simulink model "VCU_SW"  (R2020b)
settings: Solver=FixedStepDiscrete  StartTime=0.0  StopTime=inf  FixedStep=1e-2  RelTol=1e-3
PreLoadFcn:
  | RTWConfigurationCB('preloadfcn', bdroot);
InitFcn:
  | loadvar_ttc500
undefined symbols (not defined in the file or in its folder): BrkPedalTypes, CabMovModeTypes, cFuseTempSensAcc_X, cFuseTempSensAcc_Y, cFuseTempSensVal_X, cFuseTempSensVal_Y, cTMSTempSensVal_X, cTMSTempSensVal_Y, cTransferCaseSpeedRatio, diag_state, DoorsPositionTypes, dP_filter_Y, DriverOccClassSystemTypes, ErrorValueTypes, fatal_error_callback, IO_ADC_NO_RANGE, LadderStatusTypes, pAnalogCabRotSensAcc, pAnalogCabRotSensMaxVolt, pAnalogCabRotSensMinVolt, pAnalogCabRotSensRange, pAnalogCabRotSensZeroVolt, pBrkActivePress, pCabTiltSensAcc, pCabTiltSensMaxCur, pCabTiltSensMinCur, pDistanceCorrection, pECANManual_BPNEnable, pECANManual_BPNEnabler_Flag, pFilterSensAccRes, pHDirMaxDiffFrq, pHDirSensHighLvl, pHDirSensLowLvl, pMainGearRatio, pMaxFilterSensRes, pMaxFirstPedalSensValue, pMaxFuseTempSensRes, pMaxPressLoss, pMaxPressSensCurrent, pMaxPressValue, pMaxPressValueHydMotAndPump, pMaxPressValueParkDrain, pMaxSecondPedalSensValue, pMaxTempSensVoltage, pMaxTempValue, pMaxTMSTempSensRes, pMinFilterSensRes, pMinFirstPedalSensValue, pMinFuseTempSensRes, pMinPressLoss, pMinPressSensCurrent, pMinPressValue, pMinSecondPedalSensValue, pMinTempSensVoltage, pMinTempValue, pMinTMSTempSensRes, pMotorRingTeethNum, pPedalSensAccuracyPct, pPedalSensAccuracyVolt, pPressLossTreshhold ... (+20)
libraries: TTlibrary x271, canmsglib x128, simulink x88
(part 7 of 17)

== system VCU_SW/OutputLayer/OutputInterfaces/exDigitalOutput/SetDO1000msec ==
  function : TriggerPort  TriggerType=function-call  VariantControl=Variant
  Constant50 : Constant  OutDataTypeStr=uint8
  Constant51 : Constant  Value=0  OutDataTypeStr=uint8
  Data Store Read15 : DataStoreRead  DataStoreName=OutputInterfaceData  DataStoreElements=OutputInterfaceData.DO.lowBrakeFluidSensSupply
  Data Store Read61 : DataStoreRead  DataStoreName=ManualOutputInterfaceData  DataStoreElements=ManualOutputInterfaceData.DO_Man.man_lowBrakeFluidSensSupply
  Data Type Conversion25 : DataTypeConversion  OutDataTypeStr=boolean
  Function Caller16 : FunctionCaller  FunctionPrototype=rawValue = convDIOStsTypeToNum(enumValue)  InputArgumentSpecifications=<Enter example>  OutputArgumentSpecifications=<Enter example>
  Logical Operator25 : Logic  Operator=OR  AllPortsSameDT=off  OutDataTypeStr=boolean
  Multiport Switch25 : MultiPortSwitch  DataPortOrder=Zero-based contiguous  Inputs=2  zeroidx=on
  Relational Operator50 : RelationalOperator  Operator===  OutDataTypeStr=boolean  RndMeth=Simplest
  Relational Operator51 : RelationalOperator  Operator===  OutDataTypeStr=boolean  RndMeth=Simplest
  Terminator10 : Terminator
  setDigitalOutputValue16 : TTlibrary/DIO/setDigitalOutputValue  do_channel=IO_DO_41  diagnostic=FALSE  safety_conf=off  low_side_safety_channel=IO_DO_08  io_error=on  sample_time=-1
      settings: SourceProductName=TT control 500 series
  wires:
  Data Type Conversion25/1 -> Multiport Switch25/3
  Constant51/1 -> Relational Operator50/2
  Relational Operator50/1 -> Logical Operator25/2
  Multiport Switch25/1 -> setDigitalOutputValue16/1
  Logical Operator25/1 -> Multiport Switch25/1
  Data Store Read15/1 -> Function Caller16/1
  Relational Operator51/1 -> Logical Operator25/1
  Data Store Read61/1 -> Relational Operator51/1, Relational Operator50/1, Data Type Conversion25/1
  setDigitalOutputValue16/1 -> Terminator10/1
  Constant50/1 -> Relational Operator51/2
  Function Caller16/1 -> Multiport Switch25/2

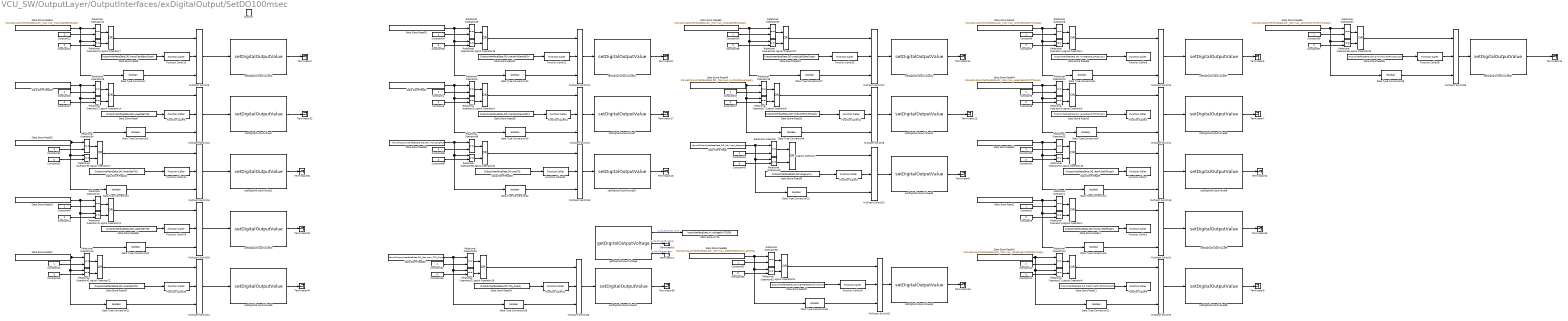
== system VCU_SW/OutputLayer/OutputInterfaces/exDigitalOutput/SetDO100msec ==
  function : TriggerPort  TriggerType=function-call  VariantControl=Variant
  Constant{2,4,6,8,10,12,16,26,30,32,34,40,42,44,52,54,56,62,68} (19 alike) : Constant  OutDataTypeStr=uint8
  Constant{3,5,7,9,11,13,17,27,31,33,35,41,43,45,53,55,57,63,69} (19 alike) : Constant  Value=0  OutDataTypeStr=uint8
  Data Store Read : DataStoreRead  DataStoreName=ManualOutputInterfaceData  DataStoreElements=ManualOutputInterfaceData.DO_Man.man_diagLamp
  Data Store Read10 : DataStoreRead  DataStoreName=OutputInterfaceData  DataStoreElements=OutputInterfaceData.DO.upperGearDistrTCSupply
  Data Store Read11 : DataStoreRead  DataStoreName=OutputInterfaceData  DataStoreElements=OutputInterfaceData.DO.disablingFrontDrDistrSupply
  Data Store Read12 : DataStoreRead  DataStoreName=OutputInterfaceData  DataStoreElements=OutputInterfaceData.DO.starterSolenoidCtrl
  Data Store Read14 : DataStoreRead  DataStoreName=OutputInterfaceData  DataStoreElements=OutputInterfaceData.DO.frontAxleDifSupply
  Data Store Read19 : DataStoreRead  DataStoreName=ManualOutputInterfaceData  DataStoreElements=ManualOutputInterfaceData.DO_Man.man_upperGenT15
  Data Store Read2 : DataStoreRead  DataStoreName=ManualOutputInterfaceData  DataStoreElements=ManualOutputInterfaceData.DO_Man.man_frontAxleDifSupply
  Data Store Read22 : DataStoreRead  DataStoreName=OutputInterfaceData  DataStoreElements=OutputInterfaceData.DO.lowerGenT15
  Data Store Read23 : DataStoreRead  DataStoreName=OutputInterfaceData  DataStoreElements=OutputInterfaceData.DO.stopLightSensSupply
  Data Store Read24 : DataStoreRead  DataStoreName=OutputInterfaceData  DataStoreElements=OutputInterfaceData.DO.lowerGenT15
  Data Store Read27 : DataStoreRead  DataStoreName=OutputInterfaceData  DataStoreElements=OutputInterfaceData.DO.engPreheaterActivationSig
  Data Store Read28 : DataStoreRead  DataStoreName=OutputInterfaceData  DataStoreElements=OutputInterfaceData.DO.starterSolenoidCtrl
  Data Store Read3 : DataStoreRead  DataStoreName=ManualOutputInterfaceData  DataStoreElements=ManualOutputInterfaceData.DO_Man.man_lowerGearDistrTCSupply
  Data Store Read31 : DataStoreRead  DataStoreName=OutputInterfaceData  DataStoreElements=OutputInterfaceData.DO.HydCANPowerSupply
  Data Store Read32 : DataStoreRead  DataStoreName=OutputInterfaceData  DataStoreElements=OutputInterfaceData.DO.engT15
  Data Store Read34 : DataStoreRead  DataStoreName=OutputInterfaceData  DataStoreElements=OutputInterfaceData.DO.T15_Supply
  Data Store Read35 : DataStoreRead  DataStoreName=OutputInterfaceData  DataStoreElements=OutputInterfaceData.DO.IgnitionSwitchPowerSupply
  Data Store Read36 : DataStoreRead  DataStoreName=OutputInterfaceData  DataStoreElements=OutputInterfaceData.DO.diagLamp
  Data Store Read39 : DataStoreRead  DataStoreName=OutputInterfaceData  DataStoreElements=OutputInterfaceData.DO.lowerGearDistrTCSupply
  Data Store Read4 : DataStoreRead  DataStoreName=ManualOutputInterfaceData  DataStoreElements=ManualOutputInterfaceData.DO_Man.man_starterSolenoidCtrl
  Data Store Read40 : DataStoreRead  DataStoreName=ManualOutputInterfaceData  DataStoreElements=ManualOutputInterfaceData.DO_Man.man_upperGearDistrTCSupply
  Data Store Read41 : DataStoreRead  DataStoreName=ManualOutputInterfaceData  DataStoreElements=ManualOutputInterfaceData.DO_Man.man_disablingFrontDrDistrSupply
  Data Store Read42 : DataStoreRead  DataStoreName=ManualOutputInterfaceData  DataStoreElements=ManualOutputInterfaceData.DO_Man.man_transCaseSensSupply
  Data Store Read44 : DataStoreRead  DataStoreName=ManualOutputInterfaceData  DataStoreElements=ManualOutputInterfaceData.DO_Man.man_HydCANPowerSupply
  Data Store Read49 : DataStoreRead  DataStoreName=ManualOutputInterfaceData  DataStoreElements=ManualOutputInterfaceData.DO_Man.man_upperGenT15
  Data Store Read5 : DataStoreRead  DataStoreName=OutputInterfaceData  DataStoreElements=OutputInterfaceData.DO.transCaseSensSupply
  Data Store Read51 : DataStoreRead  DataStoreName=ManualOutputInterfaceData  DataStoreElements=ManualOutputInterfaceData.DO_Man.man_rearAxleDifSupply
  Data Store Read52 : DataStoreRead  DataStoreName=ManualOutputInterfaceData  DataStoreElements=ManualOutputInterfaceData.DO_Man.man_lowerGenT15
  Data Store Read53 : DataStoreRead  DataStoreName=ManualOutputInterfaceData  DataStoreElements=ManualOutputInterfaceData.DO_Man.man_starterSolenoidCtrl
  Data Store Read56 : DataStoreRead  DataStoreName=OutputInterfaceData  DataStoreElements=OutputInterfaceData.DO.upperGenT15
  Data Store Read57 : DataStoreRead  DataStoreName=ManualOutputInterfaceData  DataStoreElements=ManualOutputInterfaceData.DO_Man.man_lowerGenT15
  Data Store Read62 : DataStoreRead  DataStoreName=ManualOutputInterfaceData  DataStoreElements=ManualOutputInterfaceData.DO_Man.man_T15_Supply
  Data Store Read63 : DataStoreRead  DataStoreName=ManualOutputInterfaceData  DataStoreElements=ManualOutputInterfaceData.DO_Man.man_stopLightSensSupply
  Data Store Read64 : DataStoreRead  DataStoreName=ManualOutputInterfaceData  DataStoreElements=ManualOutputInterfaceData.DO_Man.man_IgnitionSwitchPowerSupply
  Data Store Read66 : DataStoreRead  DataStoreName=ManualOutputInterfaceData  DataStoreElements=ManualOutputInterfaceData.DO_Man.man_engPreheaterActivationSig
  Data Store Read69 : DataStoreRead  DataStoreName=ManualOutputInterfaceData  DataStoreElements=ManualOutputInterfaceData.DO_Man.man_engT15
  Data Store Read7 : DataStoreRead  DataStoreName=OutputInterfaceData  DataStoreElements=OutputInterfaceData.DO.upperGenT15
  Data Store Read9 : DataStoreRead  DataStoreName=OutputInterfaceData  DataStoreElements=OutputInterfaceData.DO.rearAxleDifSupply
  Data Store Write : DataStoreWrite  DataStoreName=InputInterfaceData  DataStoreElements=InputInterfaceData.AI.voltageOnT15DO
  Data Type Conversion{,2,4..9,12..13,19..22,26..28,31,34} (19 alike) : DataTypeConversion  OutDataTypeStr=boolean
  Function Caller{1..5,7,9..13,20..21,24,26,29..31,35} (19 alike) : FunctionCaller  FunctionPrototype=rawValue = convDIOStsTypeToNum(enumValue)  InputArgumentSpecifications=<Enter example>  OutputArgumentSpecifications=<Enter example>
  Logical Operator{,1,3..7,9,14,16..18,21..22,26..28,31,34} (19 alike) : Logic  Operator=OR  AllPortsSameDT=off  OutDataTypeStr=boolean
  Multiport Switch{1..6,8,13,15..17,20..21,26..28,31,34} (18 alike) : MultiPortSwitch  DataPortOrder=Zero-based contiguous  Inputs=2  zeroidx=on
  Multiport Switch22 : MultiPortSwitch  DataPortOrder=Zero-based contiguous  Inputs=2  DiagnosticForDefault=None  zeroidx=on
  Relational Operator{,1,4..14,17..18,27..28,31..36,41..45,52..57,62..63,68..69} (38 alike) : RelationalOperator  Operator===  OutDataTypeStr=boolean  RndMeth=Simplest
  Terminator{1..3,5..9,13,16..17,32,34..36,38..39,42..44,48} (21 alike) : Terminator
  getDigitalOutputVoltage : TTlibrary/DIO/getDigitalOutputVoltage  do_channel=IO_DO_03  io_error=on  sample_time=-1
      settings: SourceProductName=TT control 500 series
  setDigitalOutputValue10 : TTlibrary/DIO/setDigitalOutputValue  do_channel=IO_DO_39  diagnostic=FALSE  safety_conf=off  low_side_safety_channel=IO_DO_08  io_error=on  sample_time=-1
      settings: SourceProductName=TT control 500 series
  setDigitalOutputValue11 : TTlibrary/DIO/setDigitalOutputValue  do_channel=IO_DO_20  diagnostic=FALSE  safety_conf=off  low_side_safety_channel=IO_DO_08  io_error=on  sample_time=-1
      settings: SourceProductName=TT control 500 series
  setDigitalOutputValue12 : TTlibrary/DIO/setDigitalOutputValue  do_channel=IO_DO_06  diagnostic=FALSE  safety_conf=off  low_side_safety_channel=IO_DO_08  io_error=on  sample_time=-1
      settings: SourceProductName=TT control 500 series
  setDigitalOutputValue13 : TTlibrary/DIO/setDigitalOutputValue  do_channel=IO_DO_45  diagnostic=FALSE  safety_conf=off  low_side_safety_channel=IO_DO_08  io_error=on  sample_time=-1
      settings: SourceProductName=TT control 500 series
  setDigitalOutputValue20 : TTlibrary/DIO/setDigitalOutputValue  do_channel=IO_DO_51  diagnostic=FALSE  safety_conf=off  low_side_safety_channel=IO_DO_08  io_error=on  sample_time=-1
      settings: SourceProductName=TT control 500 series
  setDigitalOutputValue21 : TTlibrary/DIO/setDigitalOutputValue  do_channel=IO_DO_03  diagnostic=FALSE  safety_conf=off  low_side_safety_channel=IO_DO_08  io_error=on  sample_time=-1
      settings: SourceProductName=TT control 500 series
  setDigitalOutputValue24 : TTlibrary/DIO/setDigitalOutputValue  do_channel=IO_DO_33  diagnostic=FALSE  safety_conf=off  low_side_safety_channel=IO_DO_08  io_error=on  sample_time=-1
      settings: SourceProductName=TT control 500 series
  setDigitalOutputValue25 : TTlibrary/DIO/setDigitalOutputValue  do_channel=IO_DO_07  diagnostic=FALSE  safety_conf=off  low_side_safety_channel=IO_DO_08  io_error=on  sample_time=-1
      settings: SourceProductName=TT control 500 series
  setDigitalOutputValue26 : TTlibrary/DIO/setDigitalOutputValue  do_channel=IO_DO_21  diagnostic=FALSE  safety_conf=off  low_side_safety_channel=IO_DO_08  io_error=on  sample_time=-1
      settings: SourceProductName=TT control 500 series
  setDigitalOutputValue30 : TTlibrary/DIO/setDigitalOutputValue  do_channel=IO_DO_24  diagnostic=FALSE  safety_conf=off  low_side_safety_channel=IO_DO_08  io_error=on  sample_time=-1
      settings: SourceProductName=TT control 500 series
  setDigitalOutputValue35 : TTlibrary/DIO/setDigitalOutputValue  do_channel=IO_DO_42  diagnostic=FALSE  safety_conf=off  low_side_safety_channel=IO_DO_08  io_error=on  sample_time=-1
      settings: SourceProductName=TT control 500 series
  setDigitalOutputValue36 : TTlibrary/DIO/setDigitalOutputValue  do_channel=IO_DO_34  diagnostic=FALSE  safety_conf=off  low_side_safety_channel=IO_DO_08  io_error=on  sample_time=-1
      settings: SourceProductName=TT control 500 series
  setDigitalOutputValue37 : TTlibrary/DIO/setDigitalOutputValue  do_channel=IO_DO_23  diagnostic=FALSE  safety_conf=off  low_side_safety_channel=IO_DO_08  io_error=on  sample_time=-1
      settings: SourceProductName=TT control 500 series
  setDigitalOutputValue38 : TTlibrary/DIO/setDigitalOutputValue  do_channel=IO_DO_37  diagnostic=FALSE  safety_conf=off  low_side_safety_channel=IO_DO_08  io_error=on  sample_time=-1
      settings: SourceProductName=TT control 500 series
  setDigitalOutputValue39 : TTlibrary/DIO/setDigitalOutputValue  do_channel=IO_DO_25  diagnostic=FALSE  safety_conf=off  low_side_safety_channel=IO_DO_08  io_error=on  sample_time=-1
      settings: SourceProductName=TT control 500 series
  setDigitalOutputValue4 : TTlibrary/DIO/setDigitalOutputValue  do_channel=IO_DO_50  diagnostic=FALSE  safety_conf=off  low_side_safety_channel=IO_DO_08  io_error=on  sample_time=-1
      settings: SourceProductName=TT control 500 series
  setDigitalOutputValue7 : TTlibrary/DIO/setDigitalOutputValue  do_channel=IO_DO_38  diagnostic=FALSE  safety_conf=off  low_side_safety_channel=IO_DO_08  io_error=on  sample_time=-1
      settings: SourceProductName=TT control 500 series
  setDigitalOutputValue8 : TTlibrary/DIO/setDigitalOutputValue  do_channel=IO_DO_18  diagnostic=FALSE  safety_conf=off  low_side_safety_channel=IO_DO_08  io_error=on  sample_time=-1
      settings: SourceProductName=TT control 500 series
  setDigitalOutputValue9 : TTlibrary/DIO/setDigitalOutputValue  do_channel=IO_DO_32  diagnostic=FALSE  safety_conf=off  low_side_safety_channel=IO_DO_08  io_error=on  sample_time=-1
      settings: SourceProductName=TT control 500 series
  wires:
  Logical Operator7/1 -> Multiport Switch6/1
  Multiport Switch6/1 -> setDigitalOutputValue13/1
  Function Caller13/1 -> Multiport Switch6/2
  Data Store Read5/1 -> Function Caller13/1
  Data Type Conversion/1 -> Multiport Switch6/3
  Relational Operator13/1 -> Logical Operator7/2
  setDigitalOutputValue13/1 -> Terminator2/1
  Data Store Read42/1 -> Relational Operator14/1, Relational Operator13/1, Data Type Conversion/1
  Constant13/1 -> Relational Operator13/2
  Constant12/1 -> Relational Operator14/2
  Relational Operator14/1 -> Logical Operator7/1
  Function Caller5/1 -> Multiport Switch13/2
  Constant27/1 -> Relational Operator27/2
  setDigitalOutputValue4/1 -> Terminator32/1
  Data Store Read52/1 -> Relational Operator34/1, Relational Operator33/1, Data Type Conversion7/1
  Relational Operator27/1 -> Logical Operator14/2
  Relational Operator34/1 -> Logical Operator17/1
  Constant32/1 -> Relational Operator34/2
  Constant26/1 -> Relational Operator28/2
  Relational Operator33/1 -> Logical Operator17/2
  Data Store Read49/1 -> Relational Operator28/1, Relational Operator27/1, Data Type Conversion2/1
  Function Caller10/1 -> Multiport Switch16/2
  Logical Operator17/1 -> Multiport Switch16/1
  Data Store Read22/1 -> Function Caller10/1
  Relational Operator28/1 -> Logical Operator14/1
  Data Type Conversion7/1 -> Multiport Switch16/3
  Constant33/1 -> Relational Operator33/2
  Multiport Switch13/1 -> setDigitalOutputValue4/1
  Logical Operator14/1 -> Multiport Switch13/1
  setDigitalOutputValue11/1 -> Terminator36/1
  Data Store Read7/1 -> Function Caller5/1
  Multiport Switch16/1 -> setDigitalOutputValue11/1
  Data Type Conversion2/1 -> Multiport Switch13/3
  Constant40/1 -> Relational Operator42/2
  Logical Operator21/1 -> Multiport Switch20/1
  Relational Operator42/1 -> Logical Operator21/1
  Relational Operator41/1 -> Logical Operator21/2
  Constant41/1 -> Relational Operator41/2
  Data Store Read19/1 -> Relational Operator42/1, Relational Operator41/1, Data Type Conversion20/1
  Multiport Switch20/1 -> setDigitalOutputValue20/1
  setDigitalOutputValue20/1 -> Terminator38/1
  Data Store Read56/1 -> Function Caller24/1
  Function Caller24/1 -> Multiport Switch20/2
  Data Type Conversion20/1 -> Multiport Switch20/3
  Relational Operator43/1 -> Logical Operator22/2
  Data Store Read24/1 -> Function Caller29/1
  Relational Operator44/1 -> Logical Operator22/1
  Multiport Switch21/1 -> setDigitalOutputValue26/1
  Data Type Conversion21/1 -> Multiport Switch21/3
  setDigitalOutputValue26/1 -> Terminator44/1
  Logical Operator22/1 -> Multiport Switch21/1
  Constant42/1 -> Relational Operator44/2
  Data Store Read57/1 -> Relational Operator44/1, Relational Operator43/1, Data Type Conversion21/1
  Constant43/1 -> Relational Operator43/2
  Function Caller29/1 -> Multiport Switch21/2
  Data Store Read62/1 -> Relational Operator53/1, Relational Operator52/1, Data Type Conversion26/1
  setDigitalOutputValue10/1 -> Terminator9/1
  Multiport Switch34/1 -> setDigitalOutputValue35/1
  Relational Operator36/1 -> Logical Operator18/1
  getDigitalOutputVoltage/3 -> Terminator1/1  "io_do_03_amp_error"
  Function Caller31/1 -> Multiport Switch2/2
  Data Type Conversion12/1 -> Multiport Switch17/3
  Data Store Read32/1 -> Function Caller35/1
  Logical Operator26/1 -> Multiport Switch26/1
  Multiport Switch17/1 -> setDigitalOutputValue10/1
  Data Store Read34/1 -> Function Caller21/1
  setDigitalOutputValue7/1 -> Terminator17/1
  Data Store Read12/1 -> Function Caller11/1
  Logical Operator34/1 -> Multiport Switch34/1
  Constant68/1 -> Relational Operator69/2
  Constant52/1 -> Relational Operator53/2
  Relational Operator5/1 -> Logical Operator3/2
  Function Caller11/1 -> Multiport Switch17/2
  Relational Operator52/1 -> Logical Operator26/2
  Constant53/1 -> Relational Operator52/2
  Relational Operator35/1 -> Logical Operator18/2
  Logical Operator18/1 -> Multiport Switch17/1
  getDigitalOutputVoltage/1 -> Data Store Write/1  "io_do_03_amp_value"
  setDigitalOutputValue21/1 -> Terminator39/1
  Relational Operator68/1 -> Logical Operator34/2
  Logical Operator3/1 -> Multiport Switch2/1
  Data Store Read69/1 -> Relational Operator69/1, Relational Operator68/1, Data Type Conversion34/1
  Data Store Read4/1 -> Relational Operator6/1, Relational Operator5/1, Data Type Conversion19/1
  Constant69/1 -> Relational Operator68/2
  Multiport Switch2/1 -> setDigitalOutputValue7/1
  getDigitalOutputVoltage/2 -> Terminator3/1  "io_do_03_amp_update"
  setDigitalOutputValue35/1 -> Terminator48/1
  Function Caller21/1 -> Multiport Switch26/2
  Data Type Conversion34/1 -> Multiport Switch34/3
  Data Store Read28/1 -> Function Caller31/1
  Multiport Switch26/1 -> setDigitalOutputValue21/1
  Relational Operator69/1 -> Logical Operator34/1
  Data Store Read53/1 -> Relational Operator36/1, Relational Operator35/1, Data Type Conversion12/1
  Data Type Conversion26/1 -> Multiport Switch26/3
  Constant5/1 -> Relational Operator5/2
  Constant4/1 -> Relational Operator6/2
  Data Type Conversion19/1 -> Multiport Switch2/3
  Relational Operator6/1 -> Logical Operator3/1
  Constant35/1 -> Relational Operator35/2
  Constant34/1 -> Relational Operator36/2
  Relational Operator53/1 -> Logical Operator26/1
  Function Caller35/1 -> Multiport Switch34/2
  Function Caller20/1 -> Multiport Switch27/2
  Data Type Conversion27/1 -> Multiport Switch27/3
  Constant54/1 -> Relational Operator55/2
  Logical Operator27/1 -> Multiport Switch27/1
  Constant55/1 -> Relational Operator54/2
  Relational Operator55/1 -> Logical Operator27/1
  Multiport Switch27/1 -> setDigitalOutputValue24/1
  setDigitalOutputValue24/1 -> Terminator42/1
  Data Store Read63/1 -> Relational Operator55/1, Relational Operator54/1, Data Type Conversion27/1
  Data Store Read23/1 -> Function Caller20/1
  Relational Operator54/1 -> Logical Operator27/2
  Data Store Read40/1 -> Relational Operator10/1, Relational Operator9/1, Data Type Conversion9/1
  setDigitalOutputValue37/1 -> Terminator5/1
  Data Type Conversion8/1 -> Multiport Switch3/3
  Constant11/1 -> Relational Operator11/2
  Relational Operator1/1 -> Logical Operator1/2
  Constant10/1 -> Relational Operator12/2
  Relational Operator31/1 -> Logical Operator16/2
  Data Store Read51/1 -> Relational Operator32/1, Relational Operator31/1, Data Type Conversion4/1
  Logical Operator6/1 -> Multiport Switch5/1
  Multiport Switch15/1 -> setDigitalOutputValue8/1
  setDigitalOutputValue8/1 -> Terminator34/1
  Relational Operator12/1 -> Logical Operator6/1
  setDigitalOutputValue9/1 -> Terminator35/1
  Logical Operator1/1 -> Multiport Switch1/1
  Constant3/1 -> Relational Operator1/2
  Multiport Switch5/1 -> setDigitalOutputValue39/1
  Constant31/1 -> Relational Operator31/2
  Logical Operator16/1 -> Multiport Switch15/1
  Data Store Read9/1 -> Function Caller7/1
  Relational Operator4/1 -> Logical Operator1/1
  Data Type Conversion4/1 -> Multiport Switch15/3
  Constant2/1 -> Relational Operator4/2
  Data Store Read14/1 -> Function Caller1/1
  Data Type Conversion13/1 -> Multiport Switch5/3
  Multiport Switch1/1 -> setDigitalOutputValue9/1
  setDigitalOutputValue39/1 -> Terminator8/1
  Relational Operator32/1 -> Logical Operator16/1
  Data Store Read3/1 -> Relational Operator8/1, Relational Operator7/1, Data Type Conversion8/1
  Relational Operator11/1 -> Logical Operator6/2
  Data Type Conversion5/1 -> Multiport Switch1/3
  Relational Operator7/1 -> Logical Operator4/2
  Data Store Read11/1 -> Function Caller9/1
  Constant6/1 -> Relational Operator8/2
  Constant30/1 -> Relational Operator32/2
  Multiport Switch4/1 -> setDigitalOutputValue38/1
  Data Store Read41/1 -> Relational Operator12/1, Relational Operator11/1, Data Type Conversion13/1
  setDigitalOutputValue38/1 -> Terminator7/1
  Constant9/1 -> Relational Operator9/2
  Data Store Read10/1 -> Function Caller4/1
  Logical Operator5/1 -> Multiport Switch4/1
  Multiport Switch3/1 -> setDigitalOutputValue37/1
  Relational Operator10/1 -> Logical Operator5/1
  Data Type Conversion9/1 -> Multiport Switch4/3
  Logical Operator4/1 -> Multiport Switch3/1
  Data Store Read39/1 -> Function Caller3/1
  Relational Operator9/1 -> Logical Operator5/2
  Constant8/1 -> Relational Operator10/2
  Constant7/1 -> Relational Operator7/2
  Relational Operator8/1 -> Logical Operator4/1
  Data Store Read2/1 -> Relational Operator4/1, Relational Operator1/1, Data Type Conversion5/1
  Relational Operator18/1 -> Logical Operator9/1
  Function Caller12/1 -> Multiport Switch8/2
  Data Store Read31/1 -> Function Caller12/1
  Logical Operator9/1 -> Multiport Switch8/1
  Constant17/1 -> Relational Operator17/2
  Constant16/1 -> Relational Operator18/2
  Relational Operator17/1 -> Logical Operator9/2
  setDigitalOutputValue12/1 -> Terminator13/1
  Data Type Conversion6/1 -> Multiport Switch8/3
  Data Store Read44/1 -> Relational Operator18/1, Relational Operator17/1, Data Type Conversion6/1
  Multiport Switch8/1 -> setDigitalOutputValue12/1
  Data Store Read36/1 -> Function Caller2/1
  Data Store Read/1 -> Relational Operator/1, Relational Operator45/1, Data Type Conversion22/1
  Relational Operator/1 -> Logical Operator/1
  Function Caller2/1 -> Multiport Switch22/2
  Constant44/1 -> Relational Operator/2
  setDigitalOutputValue36/1 -> Terminator6/1
  Multiport Switch22/1 -> setDigitalOutputValue36/1
  Relational Operator45/1 -> Logical Operator/2
  Logical Operator/1 -> Multiport Switch22/1
  Data Type Conversion22/1 -> Multiport Switch22/3
  Constant45/1 -> Relational Operator45/2
  Data Type Conversion31/1 -> Multiport Switch31/3
  setDigitalOutputValue30/1 -> Terminator16/1
  Function Caller26/1 -> Multiport Switch31/2
  Constant63/1 -> Relational Operator62/2
  Relational Operator63/1 -> Logical Operator31/1
  Logical Operator31/1 -> Multiport Switch31/1
  Multiport Switch31/1 -> setDigitalOutputValue30/1
  Relational Operator62/1 -> Logical Operator31/2
  Constant62/1 -> Relational Operator63/2
  Data Store Read66/1 -> Relational Operator63/1, Relational Operator62/1, Data Type Conversion31/1
  Data Store Read27/1 -> Function Caller26/1
  Function Caller30/1 -> Multiport Switch28/2
  Logical Operator28/1 -> Multiport Switch28/1
  Relational Operator56/1 -> Logical Operator28/2
  Data Type Conversion28/1 -> Multiport Switch28/3
  Data Store Read35/1 -> Function Caller30/1
  Multiport Switch28/1 -> setDigitalOutputValue25/1
  Relational Operator57/1 -> Logical Operator28/1
  Constant56/1 -> Relational Operator57/2
  Constant57/1 -> Relational Operator56/2
  Data Store Read64/1 -> Relational Operator57/1, Relational Operator56/1, Data Type Conversion28/1
  setDigitalOutputValue25/1 -> Terminator43/1

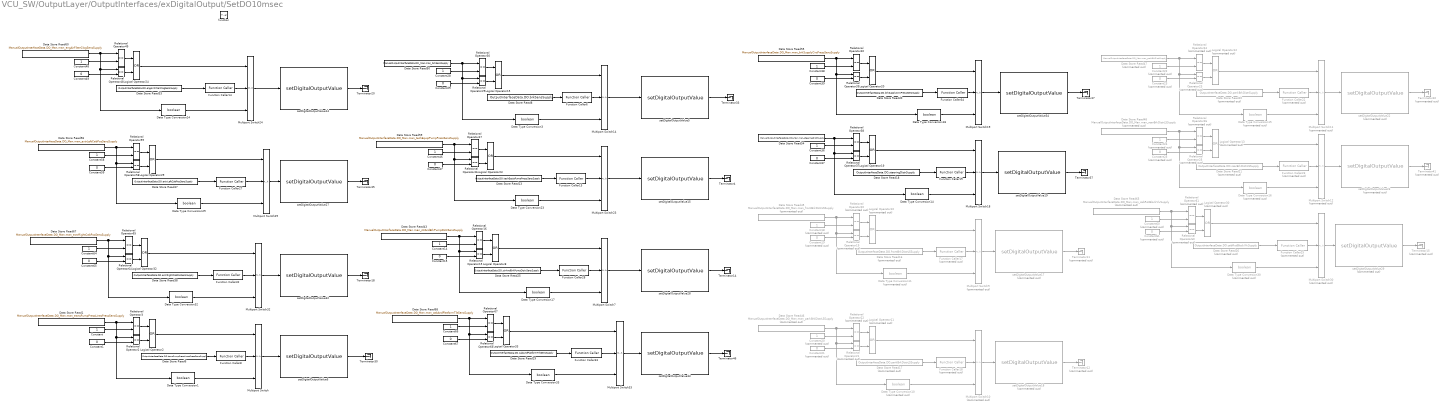
== system VCU_SW/OutputLayer/OutputInterfaces/exDigitalOutput/SetDO10msec ==
  function : TriggerPort  TriggerType=function-call  VariantControl=Variant
  Constant{,14,28,36,38,46,48,58,64,66} (10 alike) : Constant  OutDataTypeStr=uint8
  Constant{1,15,29,37,39,47,49,59,65,67} (10 alike) : Constant  Value=0  OutDataTypeStr=uint8
  Constant{18,20,22,24,60} (5 alike) : Constant  Commented=on  OutDataTypeStr=uint8
  Constant{19,21,23,25,61} (5 alike) : Constant  Commented=on  Value=0  OutDataTypeStr=uint8
  Data Store Read1 : DataStoreRead  DataStoreName=ManualOutputInterfaceData  DataStoreElements=ManualOutputInterfaceData.DO_Man.man_transPumpPressLinesPressSensSupply
  Data Store Read13 : DataStoreRead  DataStoreName=OutputInterfaceData  DataStoreElements=OutputInterfaceData.DO.techEquipPumpPressSensSupply
  Data Store Read16 : DataStoreRead  Commented=on  DataStoreName=OutputInterfaceData  DataStoreElements=OutputInterfaceData.DO.frontBrkDistrLSSupply
  Data Store Read17 : DataStoreRead  Commented=on  DataStoreName=OutputInterfaceData  DataStoreElements=OutputInterfaceData.DO.parkBrkDistrLSSupply
  Data Store Read18 : DataStoreRead  DataStoreName=OutputInterfaceData  DataStoreElements=OutputInterfaceData.DO.steeringDistrSupply
  Data Store Read20 : DataStoreRead  Commented=on  DataStoreName=OutputInterfaceData  DataStoreElements=OutputInterfaceData.DO.parkBrkDistrSupply
  Data Store Read21 : DataStoreRead  Commented=on  DataStoreName=OutputInterfaceData  DataStoreElements=OutputInterfaceData.DO.rearBrkDistrLSSupply
  Data Store Read25 : DataStoreRead  DataStoreName=OutputInterfaceData  DataStoreElements=OutputInterfaceData.DO.strAndBrkPumpDistrSensSupply
  Data Store Read26 : DataStoreRead  Commented=on  DataStoreName=OutputInterfaceData  DataStoreElements=OutputInterfaceData.DO.cabRotBlockVlvSupply
  Data Store Read29 : DataStoreRead  DataStoreName=OutputInterfaceData  DataStoreElements=OutputInterfaceData.DO.cabAndPlatformTiltSensSupply
  Data Store Read30 : DataStoreRead  DataStoreName=OutputInterfaceData  DataStoreElements=OutputInterfaceData.DO.brkSupplyCircPressSensSupply
  Data Store Read33 : DataStoreRead  DataStoreName=OutputInterfaceData  DataStoreElements=OutputInterfaceData.DO.engAirFilterClogSensSupply
  Data Store Read37 : DataStoreRead  DataStoreName=OutputInterfaceData  DataStoreElements=OutputInterfaceData.DO.extrLeftCabPosSensSupply
  Data Store Read38 : DataStoreRead  DataStoreName=OutputInterfaceData  DataStoreElements=OutputInterfaceData.DO.extrRightCabPosSensSupply
  Data Store Read43 : DataStoreRead  DataStoreName=ManualOutputInterfaceData  DataStoreElements=ManualOutputInterfaceData.DO_Man.man_strAndBrkPumpDistrSensSupply
  Data Store Read45 : DataStoreRead  Commented=on  DataStoreName=ManualOutputInterfaceData  DataStoreElements=ManualOutputInterfaceData.DO_Man.man_frontBrkDistrLSSupply
  Data Store Read46 : DataStoreRead  Commented=on  DataStoreName=ManualOutputInterfaceData  DataStoreElements=ManualOutputInterfaceData.DO_Man.man_parkBrkDistrLSSupply
  Data Store Read47 : DataStoreRead  Commented=on  DataStoreName=ManualOutputInterfaceData  DataStoreElements=ManualOutputInterfaceData.DO_Man.man_parkBrkDistrSupply
  Data Store Read48 : DataStoreRead  Commented=on  DataStoreName=ManualOutputInterfaceData  DataStoreElements=ManualOutputInterfaceData.DO_Man.man_rearBrkDistrLSSupply
  Data Store Read50 : DataStoreRead  DataStoreName=ManualOutputInterfaceData  DataStoreElements=ManualOutputInterfaceData.DO_Man.man_brkSensSupply
  Data Store Read54 : DataStoreRead  DataStoreName=ManualOutputInterfaceData  DataStoreElements=ManualOutputInterfaceData.DO_Man.man_steeringDistrSupply
  Data Store Read55 : DataStoreRead  DataStoreName=ManualOutputInterfaceData  DataStoreElements=ManualOutputInterfaceData.DO_Man.man_brkSupplyCircPressSensSupply
  Data Store Read58 : DataStoreRead  DataStoreName=ManualOutputInterfaceData  DataStoreElements=ManualOutputInterfaceData.DO_Man.man_extrLeftCabPosSensSupply
  Data Store Read59 : DataStoreRead  DataStoreName=ManualOutputInterfaceData  DataStoreElements=ManualOutputInterfaceData.DO_Man.man_techEquipPumpPressSensSupply
  Data Store Read6 : DataStoreRead  DataStoreName=OutputInterfaceData  DataStoreElements=OutputInterfaceData.DO.transPumpPressLinesPressSensSupply
  Data Store Read60 : DataStoreRead  DataStoreName=ManualOutputInterfaceData  DataStoreElements=ManualOutputInterfaceData.DO_Man.man_engAirFilterClogSensSupply
  Data Store Read65 : DataStoreRead  Commented=on  DataStoreName=ManualOutputInterfaceData  DataStoreElements=ManualOutputInterfaceData.DO_Man.man_cabRotBlockVlvSupply
  Data Store Read67 : DataStoreRead  DataStoreName=ManualOutputInterfaceData  DataStoreElements=ManualOutputInterfaceData.DO_Man.man_extrRightCabPosSensSupply
  Data Store Read68 : DataStoreRead  DataStoreName=ManualOutputInterfaceData  DataStoreElements=ManualOutputInterfaceData.DO_Man.man_cabAndPlatformTiltSensSupply
  Data Store Read8 : DataStoreRead  DataStoreName=OutputInterfaceData  DataStoreElements=OutputInterfaceData.DO.brkSensSupply
  Data Type Conversion{1,3,14,17..18,23..24,29,32..33} (10 alike) : DataTypeConversion  OutDataTypeStr=boolean
  Data Type Conversion{10..11,15..16,30} (5 alike) : DataTypeConversion  Commented=on  OutDataTypeStr=boolean
  Function Caller{6,8,14..15,19,27..28,32..34} (10 alike) : FunctionCaller  FunctionPrototype=rawValue = convDIOStsTypeToNum(enumValue)  InputArgumentSpecifications=<Enter example>  OutputArgumentSpecifications=<Enter example>
  Function Caller{17..18,22..23,25} (5 alike) : FunctionCaller  Commented=on  FunctionPrototype=rawValue = convDIOStsTypeToNum(enumValue)  InputArgumentSpecifications=<Enter example>  OutputArgumentSpecifications=<Enter example>
  Logical Operator{10..13,30} (5 alike) : Logic  Commented=on  Operator=OR  AllPortsSameDT=off  OutDataTypeStr=boolean
  Logical Operator{2,8,15,19..20,23..24,29,32..33} (10 alike) : Logic  Operator=OR  AllPortsSameDT=off  OutDataTypeStr=boolean
  Multiport Switch{,7,14,18..19,23..24,29,32..33} (10 alike) : MultiPortSwitch  DataPortOrder=Zero-based contiguous  Inputs=2  zeroidx=on
  Multiport Switch{9..12,30} (5 alike) : MultiPortSwitch  Commented=on  DataPortOrder=Zero-based contiguous  Inputs=2  zeroidx=on
  Relational Operator{2..3,15..16,29..30,37..40,46..49,58..59,64..67} (20 alike) : RelationalOperator  Operator===  OutDataTypeStr=boolean  RndMeth=Simplest
  Relational Operator{19..26,60..61} (10 alike) : RelationalOperator  Commented=on  Operator===  OutDataTypeStr=boolean  RndMeth=Simplest
  Terminator{11..12,15,40..41} (5 alike) : Terminator  Commented=on
  Terminator{4,14,18,20,30,33,37,45..47} (10 alike) : Terminator
  setDigitalOutputValue14 : TTlibrary/DIO/setDigitalOutputValue  do_channel=IO_DO_55  diagnostic=FALSE  safety_conf=off  low_side_safety_channel=IO_DO_08  io_error=on  sample_time=-1
      settings: SourceProductName=TT control 500 series
  setDigitalOutputValue15 : TTlibrary/DIO/setDigitalOutputValue  do_channel=IO_DO_27  diagnostic=FALSE  safety_conf=off  low_side_safety_channel=IO_DO_08  io_error=on  sample_time=-1
      settings: SourceProductName=TT control 500 series
  setDigitalOutputValue17 : TTlibrary/DIO/setDigitalOutputValue  Commented=on  do_channel=IO_DO_29  diagnostic=FALSE  safety_conf=off  low_side_safety_channel=IO_DO_08  io_error=on  sample_time=-1
      settings: SourceProductName=TT control 500 series
  setDigitalOutputValue18 : TTlibrary/DIO/setDigitalOutputValue  Commented=on  do_channel=IO_DO_43  diagnostic=FALSE  safety_conf=off  low_side_safety_channel=IO_DO_08  io_error=on  sample_time=-1
      settings: SourceProductName=TT control 500 series
  setDigitalOutputValue19 : TTlibrary/DIO/setDigitalOutputValue  do_channel=IO_DO_47  diagnostic=FALSE  safety_conf=off  low_side_safety_channel=IO_DO_08  io_error=on  sample_time=-1
      settings: SourceProductName=TT control 500 series
  setDigitalOutputValue22 : TTlibrary/DIO/setDigitalOutputValue  Commented=on  do_channel=IO_DO_17  diagnostic=FALSE  safety_conf=off  low_side_safety_channel=IO_DO_08  io_error=on  sample_time=-1
      settings: SourceProductName=TT control 500 series
  setDigitalOutputValue23 : TTlibrary/DIO/setDigitalOutputValue  Commented=on  do_channel=IO_DO_31  diagnostic=FALSE  safety_conf=off  low_side_safety_channel=IO_DO_08  io_error=on  sample_time=-1
      settings: SourceProductName=TT control 500 series
  setDigitalOutputValue27 : TTlibrary/DIO/setDigitalOutputValue  do_channel=IO_DO_53  diagnostic=FALSE  safety_conf=off  low_side_safety_channel=IO_DO_08  io_error=on  sample_time=-1
      settings: SourceProductName=TT control 500 series
  setDigitalOutputValue28 : TTlibrary/DIO/setDigitalOutputValue  do_channel=IO_DO_22  diagnostic=FALSE  safety_conf=off  low_side_safety_channel=IO_DO_08  io_error=on  sample_time=-1
      settings: SourceProductName=TT control 500 series
  setDigitalOutputValue29 : TTlibrary/DIO/setDigitalOutputValue  Commented=on  do_channel=IO_DO_36  diagnostic=FALSE  safety_conf=off  low_side_safety_channel=IO_DO_08  io_error=on  sample_time=-1
      settings: SourceProductName=TT control 500 series
  setDigitalOutputValue32 : TTlibrary/DIO/setDigitalOutputValue  do_channel=IO_DO_56  diagnostic=FALSE  safety_conf=off  low_side_safety_channel=IO_DO_08  io_error=on  sample_time=-1
      settings: SourceProductName=TT control 500 series
  setDigitalOutputValue33 : TTlibrary/DIO/setDigitalOutputValue  do_channel=IO_DO_26  diagnostic=FALSE  safety_conf=off  low_side_safety_channel=IO_DO_08  io_error=on  sample_time=-1
      settings: SourceProductName=TT control 500 series
  setDigitalOutputValue34 : TTlibrary/DIO/setDigitalOutputValue  do_channel=IO_DO_40  diagnostic=FALSE  safety_conf=off  low_side_safety_channel=IO_DO_08  io_error=on  sample_time=-1
      settings: SourceProductName=TT control 500 series
  setDigitalOutputValue5 : TTlibrary/DIO/setDigitalOutputValue  do_channel=IO_DO_16  diagnostic=FALSE  safety_conf=off  low_side_safety_channel=IO_DO_08  io_error=on  sample_time=-1
      settings: SourceProductName=TT control 500 series
  setDigitalOutputValue6 : TTlibrary/DIO/setDigitalOutputValue  do_channel=IO_DO_46  diagnostic=FALSE  safety_conf=off  low_side_safety_channel=IO_DO_08  io_error=on  sample_time=-1
      settings: SourceProductName=TT control 500 series
  wires:
  Multiport Switch24/1 -> setDigitalOutputValue14/1
  Function Caller14/1 -> Multiport Switch24/2
  Relational Operator48/1 -> Logical Operator24/2
  Logical Operator24/1 -> Multiport Switch24/1
  Constant48/1 -> Relational Operator49/2
  Data Store Read60/1 -> Relational Operator49/1, Relational Operator48/1, Data Type Conversion24/1
  Relational Operator49/1 -> Logical Operator24/1
  Constant49/1 -> Relational Operator48/2
  Data Type Conversion24/1 -> Multiport Switch24/3
  Data Store Read33/1 -> Function Caller14/1
  setDigitalOutputValue14/1 -> Terminator20/1
  Data Store Read58/1 -> Relational Operator59/1, Relational Operator58/1, Data Type Conversion29/1
  Relational Operator58/1 -> Logical Operator29/2
  Multiport Switch29/1 -> setDigitalOutputValue27/1
  Relational Operator59/1 -> Logical Operator29/1
  Data Store Read37/1 -> Function Caller27/1
  setDigitalOutputValue27/1 -> Terminator45/1
  Constant58/1 -> Relational Operator59/2
  Function Caller27/1 -> Multiport Switch29/2
  Constant59/1 -> Relational Operator58/2
  Data Type Conversion29/1 -> Multiport Switch29/3
  Logical Operator29/1 -> Multiport Switch29/1
  Logical Operator32/1 -> Multiport Switch32/1
  Function Caller32/1 -> Multiport Switch32/2
  setDigitalOutputValue32/1 -> Terminator18/1
  Data Store Read38/1 -> Function Caller32/1
  Data Store Read67/1 -> Relational Operator65/1, Relational Operator64/1, Data Type Conversion32/1
  Constant65/1 -> Relational Operator64/2
  Relational Operator64/1 -> Logical Operator32/2
  Multiport Switch32/1 -> setDigitalOutputValue32/1
  Data Type Conversion32/1 -> Multiport Switch32/3
  Relational Operator65/1 -> Logical Operator32/1
  Constant64/1 -> Relational Operator65/2
  Logical Operator2/1 -> Multiport Switch/1
  Multiport Switch/1 -> setDigitalOutputValue6/1
  Relational Operator3/1 -> Logical Operator2/1
  Data Store Read1/1 -> Relational Operator3/1, Relational Operator2/1, Data Type Conversion1/1
  Data Type Conversion1/1 -> Multiport Switch/3
  Relational Operator2/1 -> Logical Operator2/2
  Constant/1 -> Relational Operator3/2
  Data Store Read6/1 -> Function Caller8/1
  setDigitalOutputValue6/1 -> Terminator30/1
  Function Caller8/1 -> Multiport Switch/2
  Constant1/1 -> Relational Operator2/2
  Data Store Read13/1 -> Function Caller15/1
  Constant47/1 -> Relational Operator46/2
  Function Caller15/1 -> Multiport Switch23/2
  Logical Operator23/1 -> Multiport Switch23/1
  Data Type Conversion23/1 -> Multiport Switch23/3
  Data Store Read59/1 -> Relational Operator47/1, Relational Operator46/1, Data Type Conversion23/1
  Relational Operator47/1 -> Logical Operator23/1
  Relational Operator46/1 -> Logical Operator23/2
  Multiport Switch23/1 -> setDigitalOutputValue15/1
  setDigitalOutputValue15/1 -> Terminator4/1
  Constant46/1 -> Relational Operator47/2
  Data Type Conversion17/1 -> Multiport Switch7/3
  Constant14/1 -> Relational Operator16/2
  Data Store Read25/1 -> Function Caller28/1
  Multiport Switch7/1 -> setDigitalOutputValue28/1
  Function Caller28/1 -> Multiport Switch7/2
  Data Store Read43/1 -> Relational Operator16/1, Relational Operator15/1, Data Type Conversion17/1
  setDigitalOutputValue28/1 -> Terminator14/1
  Logical Operator8/1 -> Multiport Switch7/1
  Relational Operator15/1 -> Logical Operator8/2
  Constant15/1 -> Relational Operator15/2
  Relational Operator16/1 -> Logical Operator8/1
  Relational Operator39/1 -> Logical Operator20/2
  Relational Operator67/1 -> Logical Operator33/1
  Multiport Switch33/1 -> setDigitalOutputValue33/1
  Relational Operator40/1 -> Logical Operator20/1
  Logical Operator33/1 -> Multiport Switch33/1
  Relational Operator66/1 -> Logical Operator33/2
  Data Store Read68/1 -> Relational Operator67/1, Relational Operator66/1, Data Type Conversion33/1
  Logical Operator20/1 -> Multiport Switch19/1
  Data Type Conversion33/1 -> Multiport Switch33/3
  setDigitalOutputValue33/1 -> Terminator46/1
  Constant38/1 -> Relational Operator40/2
  Constant66/1 -> Relational Operator67/2
  Data Store Read55/1 -> Relational Operator40/1, Relational Operator39/1, Data Type Conversion18/1
  Constant39/1 -> Relational Operator39/2
  Multiport Switch19/1 -> setDigitalOutputValue34/1
  Data Store Read29/1 -> Function Caller33/1
  Function Caller33/1 -> Multiport Switch33/2
  Constant67/1 -> Relational Operator66/2
  Data Store Read30/1 -> Function Caller34/1
  Data Type Conversion18/1 -> Multiport Switch19/3
  setDigitalOutputValue34/1 -> Terminator47/1
  Function Caller34/1 -> Multiport Switch19/2
  Relational Operator37/1 -> Logical Operator19/2
  Logical Operator19/1 -> Multiport Switch18/1
  Constant37/1 -> Relational Operator37/2
  Data Type Conversion14/1 -> Multiport Switch18/3
  setDigitalOutputValue19/1 -> Terminator37/1
  Constant36/1 -> Relational Operator38/2
  Multiport Switch18/1 -> setDigitalOutputValue19/1
  Data Store Read18/1 -> Function Caller19/1
  Relational Operator38/1 -> Logical Operator19/1
  Data Store Read54/1 -> Relational Operator38/1, Relational Operator37/1, Data Type Conversion14/1
  Function Caller19/1 -> Multiport Switch18/2
  Data Type Conversion3/1 -> Multiport Switch14/3
  Multiport Switch14/1 -> setDigitalOutputValue5/1
  Constant28/1 -> Relational Operator30/2
  Constant29/1 -> Relational Operator29/2
  Logical Operator15/1 -> Multiport Switch14/1
  Data Store Read50/1 -> Relational Operator30/1, Relational Operator29/1, Data Type Conversion3/1
  Data Store Read8/1 -> Function Caller6/1
  setDigitalOutputValue5/1 -> Terminator33/1
  Relational Operator29/1 -> Logical Operator15/2
  Relational Operator30/1 -> Logical Operator15/1
  Function Caller6/1 -> Multiport Switch14/2
  Relational Operator19/1 -> Logical Operator10/2
  Logical Operator10/1 -> Multiport Switch9/1
  setDigitalOutputValue17/1 -> Terminator11/1
  Constant20/1 -> Relational Operator22/2
  Data Store Read17/1 -> Function Caller18/1
  Relational Operator21/1 -> Logical Operator11/2
  setDigitalOutputValue18/1 -> Terminator12/1
  Multiport Switch9/1 -> setDigitalOutputValue17/1
  Relational Operator22/1 -> Logical Operator11/1
  Data Store Read16/1 -> Function Caller17/1
  Constant19/1 -> Relational Operator19/2
  Logical Operator11/1 -> Multiport Switch10/1
  Constant21/1 -> Relational Operator21/2
  Multiport Switch10/1 -> setDigitalOutputValue18/1
  Relational Operator20/1 -> Logical Operator10/1
  Data Type Conversion10/1 -> Multiport Switch10/3
  Data Type Conversion11/1 -> Multiport Switch9/3
  Function Caller17/1 -> Multiport Switch9/2
  Function Caller18/1 -> Multiport Switch10/2
  Constant18/1 -> Relational Operator20/2
  Data Store Read45/1 -> Relational Operator20/1, Relational Operator19/1, Data Type Conversion11/1
  Data Store Read46/1 -> Relational Operator22/1, Relational Operator21/1, Data Type Conversion10/1
  Constant22/1 -> Relational Operator24/2
  Constant23/1 -> Relational Operator23/2
  Multiport Switch12/1 -> setDigitalOutputValue23/1
  Data Store Read47/1 -> Relational Operator24/1, Relational Operator23/1, Data Type Conversion15/1
  Relational Operator24/1 -> Logical Operator12/1
  Data Type Conversion15/1 -> Multiport Switch11/3
  Data Store Read21/1 -> Function Caller23/1
  Multiport Switch11/1 -> setDigitalOutputValue22/1
  setDigitalOutputValue23/1 -> Terminator41/1
  Constant25/1 -> Relational Operator25/2
  Data Type Conversion16/1 -> Multiport Switch12/3
  Logical Operator13/1 -> Multiport Switch12/1
  Data Store Read48/1 -> Relational Operator26/1, Relational Operator25/1, Data Type Conversion16/1
  Function Caller22/1 -> Multiport Switch11/2
  Relational Operator25/1 -> Logical Operator13/2
  Function Caller23/1 -> Multiport Switch12/2
  Constant24/1 -> Relational Operator26/2
  Relational Operator23/1 -> Logical Operator12/2
  Relational Operator26/1 -> Logical Operator13/1
  Logical Operator12/1 -> Multiport Switch11/1
  setDigitalOutputValue22/1 -> Terminator40/1
  Data Store Read20/1 -> Function Caller22/1
  Data Store Read65/1 -> Relational Operator61/1, Relational Operator60/1, Data Type Conversion30/1
  setDigitalOutputValue29/1 -> Terminator15/1
  Logical Operator30/1 -> Multiport Switch30/1
  Constant60/1 -> Relational Operator61/2
  Relational Operator60/1 -> Logical Operator30/2
  Function Caller25/1 -> Multiport Switch30/2
  Data Store Read26/1 -> Function Caller25/1
  Multiport Switch30/1 -> setDigitalOutputValue29/1
  Constant61/1 -> Relational Operator60/2
  Data Type Conversion30/1 -> Multiport Switch30/3
  Relational Operator61/1 -> Logical Operator30/1

== system VCU_SW/OutputLayer/OutputNetwork/OutputCCAN/SetCCAN1000msec ==
  function : TriggerPort  TriggerType=function-call  VariantControl=Variant
  CANPack_DCDC_IN_Control : canmsglib/CAN Pack  Commented=on  CANdbFile=C:\Users\shevchenko\Desktop\HerculesLittle\HerculesLittle\database\ElectricCAN.dbc  MsgList=(none)  MsgName=DCDC_IN_Control  MsgIDType=Extended (29-bit identifier)  MsgIdentifier=73  MsgLength=8  Remote=off  ApplyMinMax=off  BusOutput=on  SignalInfo={'BPN_Enable','0','1','LE','unsigned','Standard','0','1','0','0','1'}
      settings: SourceProductBaseCode=ME,XP,VN  DataFormat=CANdb specified signals
  CANPack_DCDC_IN_Control1 : canmsglib/CAN Pack  Commented=on  MsgList=(none)  MsgName=ETC2  MsgIDType=Extended (29-bit identifier)  MsgIdentifier=418383354  MsgLength=8  Remote=off  ApplyMinMax=off  BusOutput=on  SignalInfo={ 'Transmission_Actual_Gear_Ratio', '8', '16', 'LE', 'unsigned', 'Standard', '0', '0.001', '0', '0', '64.255'; 'Transmission_Current_Gear', '24', '8', 'LE', 'unsigned', 'Standard', '0', '1', '-125', '-125', '125'; 'Transmission_Current_Range', '48', '16', 'LE', 'unsigned', 'Standard', '0', '1', '0', '0', '65535'; 'Transmission_Requested_Range', '32', '16', 'LE', 'unsigned', 'Standard', '0', '1', '0', '0', '65535'; 'Transmission_Selected_Gear', '0', '8', 'LE', 'unsigned', 'Standard', '0', '1', '-125', '-125', '125' }
      settings: SourceProductBaseCode=ME,XP,VN  DataFormat=manually specified signals
  Constant31 : Constant  Commented=on  Value=pECANManual_BPNEnabler_Flag
  Constant32 : Constant  Commented=on  Value=pECANManual_BPNEnable
  DD_VCU : Subsystem
  DLCC1 : Subsystem
  "DLCC2 " : Subsystem
  Data Store Read : DataStoreRead  Commented=on  DataStoreName=OutputNetworkData  DataStoreElements=DevicesControllerData.ovc_permission
  Data Store Read1 : DataStoreRead  Commented=on  DataStoreName=OutputNetworkData  DataStoreElements=DevicesControllerData.ovc_permission
  "ET1 " : Subsystem
  Eletcric_current_info : Subsystem
  Eletcric_info : Subsystem
  HTR : Subsystem
  Hyd_transm_info : Subsystem
  Hyd_transm_speed_info : Subsystem
  LCMD : Subsystem
  MATLAB Function6 : MATLAB Function  Commented=on  TreatAsAtomicUnit=on
  MTUInformationArea : Subsystem
  Multiport Switch5 : MultiPortSwitch  Commented=on  DataPortOrder=Zero-based contiguous  Inputs=2  zeroidx=on
  TCI : Subsystem
  TRF2 : Subsystem
  Terminator : Terminator  Commented=on
  Terminator1 : Terminator  Commented=on
  VH : Subsystem
  transmit_message_dcdc_in_control : TTlibrary/CAN/transmit_message_name  Commented=on  channel=IO_CAN_CHANNEL_0  id_format=IO_CAN_STD_FRAME  retranslation=off  io_error=on  sample_time=-1
      settings: SourceProductName=TT control 500 series
  transmit_message_dcdc_in_control1 : TTlibrary/CAN/transmit_message_name  Commented=on  channel=IO_CAN_CHANNEL_1  id_format=IO_CAN_STD_FRAME  retranslation=off  io_error=on  sample_time=-1
      settings: SourceProductName=TT control 500 series
  wires:
  transmit_message_dcdc_in_control1/1 -> Terminator1/1  "error_tx_transmit_message_dcdc_in_control1"
  Data Store Read1/1 -> CANPack_DCDC_IN_Control1/1
  CANPack_DCDC_IN_Control1/1 -> transmit_message_dcdc_in_control1/1
  Data Store Read/1 -> MATLAB Function6/1(input)
  transmit_message_dcdc_in_control/1 -> Terminator/1  "error_tx_transmit_message_dcdc_in_control"
  MATLAB Function6/1(value) -> Multiport Switch5/2
  Multiport Switch5/1 -> CANPack_DCDC_IN_Control/1
  Constant32/1 -> Multiport Switch5/3
  CANPack_DCDC_IN_Control/1 -> transmit_message_dcdc_in_control/1
  Constant31/1 -> Multiport Switch5/1
